simulink model "modular_Lin_Modell_test"  (R2016b)
settings: Solver=VariableStepAuto  StartTime=0.0  StopTime=300  RelTol=1e-3
values from neighbouring files (symbols this model uses):
  st1 = 1    [modell_parameter.m]
settings Model: Creator=Fritz  LastModifiedBy=Fritz

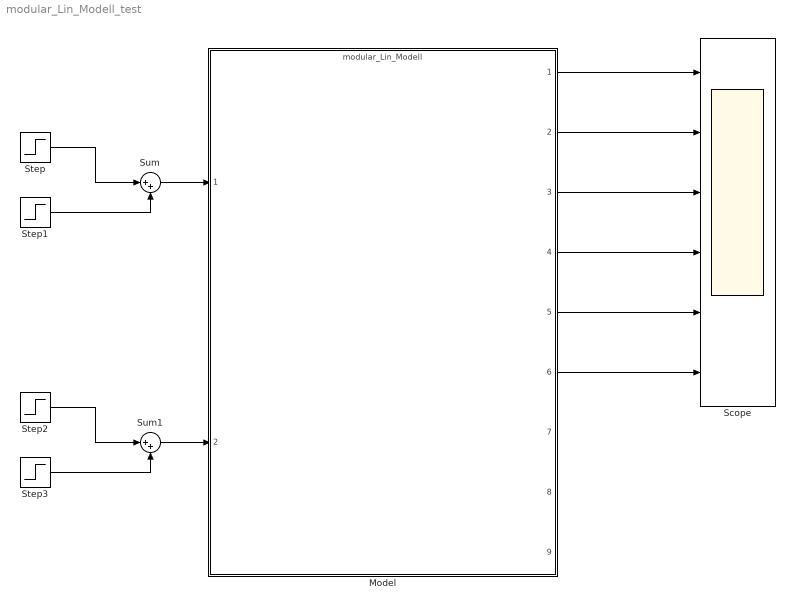
== system modular_Lin_Modell_test ==
  Model : ModelReference  ModelNameDialog=modular_Lin_Modell.slx  SimulationMode=Normal  ModelReferenceVersion=1.30
  Scope : Scope  NumInputPorts=6
  Step : Step  After=st1  SampleTime=0
  Step1 : Step  Time=10  After=-st1  SampleTime=0
  Step2 : Step  Time=10  After=0.1  SampleTime=0
  Step3 : Step  Time=15  After=-0.1  SampleTime=0
  Sum : Sum  Inputs=|++
  Sum1 : Sum  Inputs=|++
  wires:
  Model/1 -> Scope/1
  Model/2 -> Scope/2
  Model/3 -> Scope/3
  Model/4 -> Scope/4
  Model/5 -> Scope/5
  Model/6 -> Scope/6
  Step/1 -> Sum/1
  Step1/1 -> Sum/2
  Step2/1 -> Sum1/1
  Step3/1 -> Sum1/2
  Sum/1 -> Model/1
  Sum1/1 -> Model/2
